simulink model "Multiplexer8To1Circuit"  (R2023a)
settings: Solver=VariableStepAuto  StartTime=0.0  StopTime=1  RelTol=1e-3
settings Model: Creator=Admin  LastModifiedBy=Admin

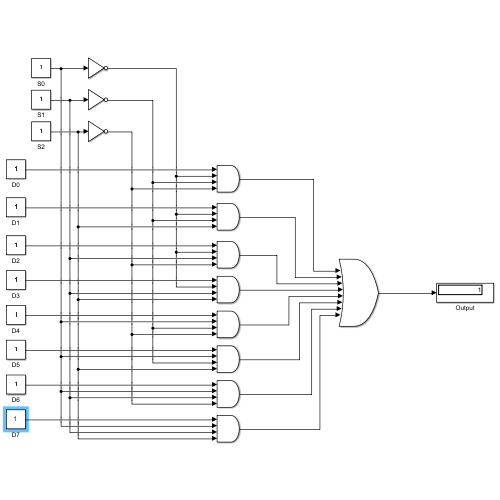
[thumbnail: Simulink's stored preview of the top-level diagram]
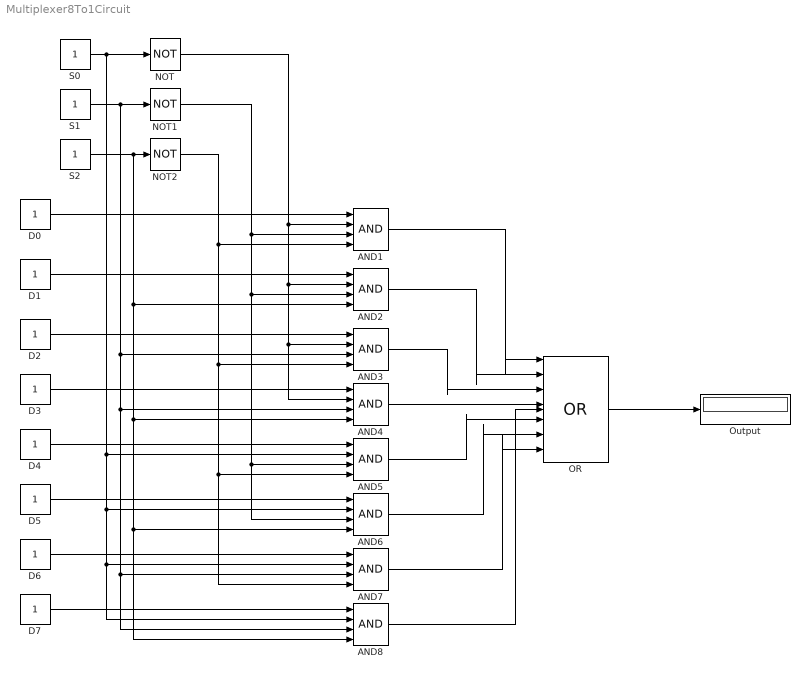
== system Multiplexer8To1Circuit ==
  AND{1..8} (8 alike) : Logic  Inputs=4  IconShape=distinctive  AllPortsSameDT=off  OutDataTypeStr=boolean
  D{0..7} (8 alike) : Constant  SampleTime=-1
  NOT : Logic  Operator=NOT  IconShape=distinctive  AllPortsSameDT=off  OutDataTypeStr=boolean
  NOT1 : Logic  Operator=NOT  IconShape=distinctive  AllPortsSameDT=off  OutDataTypeStr=boolean
  NOT2 : Logic  Operator=NOT  IconShape=distinctive  AllPortsSameDT=off  OutDataTypeStr=boolean
  OR : Logic  Operator=OR  Inputs=8  IconShape=distinctive  AllPortsSameDT=off  OutDataTypeStr=boolean
  Output : Display
  S0 : Constant  SampleTime=-1
  S1 : Constant  SampleTime=-1
  S2 : Constant  SampleTime=-1
  wires:
  S0/1 -> AND5/2, AND6/2, AND7/2, AND8/2, NOT/1
  S1/1 -> AND3/3, AND4/3, AND7/3, AND8/3, NOT1/1
  S2/1 -> AND2/4, AND4/4, AND6/4, AND8/4, NOT2/1
  NOT/1 -> AND1/2, AND2/2, AND3/2, AND4/2
  NOT1/1 -> AND1/3, AND2/3, AND5/3, AND6/3
  NOT2/1 -> AND1/4, AND3/4, AND5/4, AND7/4
  D0/1 -> AND1/1
  D1/1 -> AND2/1
  D2/1 -> AND3/1
  D3/1 -> AND4/1
  D4/1 -> AND5/1
  D5/1 -> AND6/1
  D6/1 -> AND7/1
  D7/1 -> AND8/1
  AND1/1 -> OR/1
  AND2/1 -> OR/2
  AND3/1 -> OR/3
  AND4/1 -> OR/4
  AND5/1 -> OR/5
  AND6/1 -> OR/6
  AND7/1 -> OR/7
  AND8/1 -> OR/8
  OR/1 -> Output/1
